simulink model "test3_2_model"  (R2018b)
settings: Solver=VariableStepAuto  StartTime=0.0  StopTime=Endtime  RelTol=1e-3
values from neighbouring files (symbols this model uses):
  C = 100e-6    (= 0.0001)    [test3_2.m]
  L = 100e-3    (= 0.1)    [test3_2.m]
  R = 100    [test3_2.m]
  smp = 0.001    [test3_2.m]
  V = 5    [test3_2.m]
settings Model: Creator=nharada  LastModifiedBy=nharada

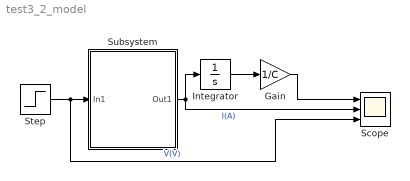
== system test3_2_model ==
  Gain : Gain  Gain=1/C
  Integrator : Integrator
  Scope : Scope  NumInputPorts=3
  Step : Step  Time=0.1  After=V  SampleTime=smp
  Subsystem : Subsystem
  wires:
  Step/1 -> Scope/3, Subsystem/1(In1)  "V(V)"
  Subsystem/1(Out1) -> Integrator/1, Scope/2  "I(A)"
  Gain/1 -> Scope/1
  Integrator/1 -> Gain/1

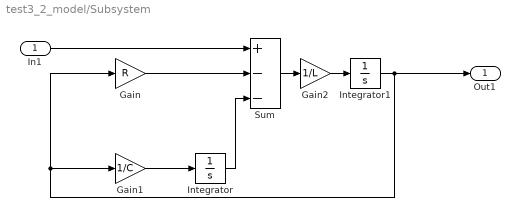
== system test3_2_model/Subsystem ==
  In1 : Inport
  Gain : Gain  Gain=R
  Gain1 : Gain  Gain=1/C
  Gain2 : Gain  Gain=1/L
  Integrator : Integrator
  Integrator1 : Integrator
  Sum : Sum  Inputs=+--
  Out1 : Outport
  wires:
  Integrator1/1 -> Gain/1, Gain1/1, Out1/1
  Integrator/1 -> Sum/3
  Gain1/1 -> Integrator/1
  Sum/1 -> Gain2/1
  Gain/1 -> Sum/2
  Gain2/1 -> Integrator1/1
  In1/1 -> Sum/1
